simulink model "sim_6a"  (R2022b)
settings: Solver=FixedStepAuto  StartTime=0.0  StopTime=240  FixedStep=10  RelTol=1e-3
values from neighbouring files (symbols this model uses):
  a1 = -0.0583    [identa2sek.m]
  b1 = 0.0074    [identa2sek.m]
  b2 = -5.4078e-06    [identa2sek.m]
settings Model: Creator=DFUNDO  LastModifiedBy=DFUNDO

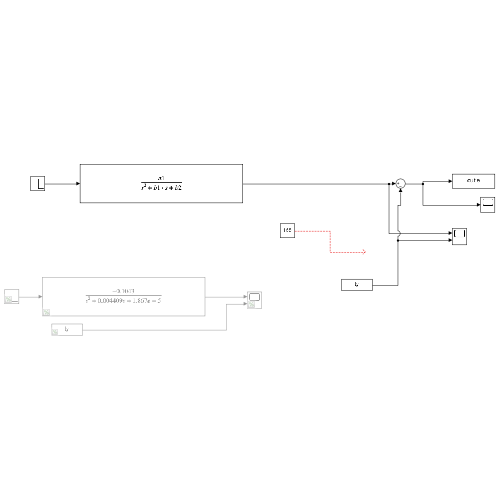
[thumbnail: Simulink's stored preview of the top-level diagram]
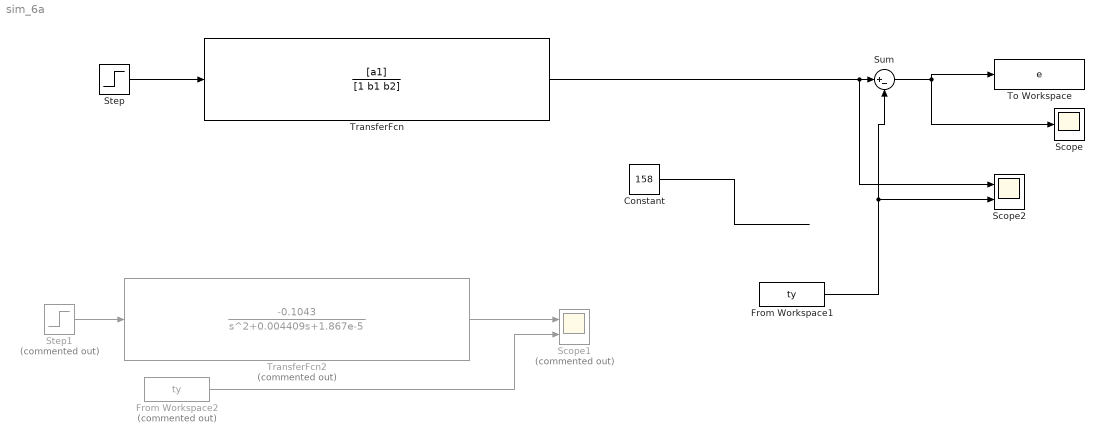
== system sim_6a ==
  Constant : Constant  Value=158
  From Workspace1 : FromWorkspace  VariableName=ty
  From Workspace2 : FromWorkspace  Commented=on  VariableName=ty
  Scope : Scope
  Scope1 : Scope  Commented=on  NumInputPorts=2
  Scope2 : Scope  NumInputPorts=2
  Step : Step  Time=10  Before=1  After=0  SampleTime=10
  Step1 : Step  Commented=on  Time=10  Before=1  After=0  SampleTime=10
  Sum : Sum  Inputs=|+-
  To Workspace : ToWorkspace  VariableName=e  SampleTime=-1
      settings: Save2DSignal=2-D array (concatenate along first dimension)
  TransferFcn : TransferFcn  Numerator=[a1]  Denominator=[1 b1 b2]
  TransferFcn2 : TransferFcn  Commented=on  Numerator=[-0.1043]  Denominator=[1 0.004409 1.867e-5]
  wires:
  Step/1 -> TransferFcn/1
  From Workspace1/1 -> Sum/2, Scope2/2
  Sum/1 -> Scope/1, To Workspace/1
  TransferFcn/1 -> Scope2/1, Sum/1
  Constant/1 -> ?
  Step1/1 -> TransferFcn2/1
  TransferFcn2/1 -> Scope1/1
  From Workspace2/1 -> Scope1/2
